simulink model "controller"  (R2019b)
settings: Solver=VariableStepAuto  StartTime=0.0  StopTime=10.0  RelTol=1e-3
undefined symbols (not defined in the file): maxPow1, maxPow2, maxPow3, maxTemp1, maxTemp2, maxTemp3, minTemp1, minTemp2, minTemp3, Pow1, Pow2, Pow3, Temp1, Temp2, Temp3
settings Model: Creator=wiart1  LastModifiedBy=tparis
settings DataIOCC: SaveFinalState=on  SaveOperatingPoint=on  SaveFormat=StructureWithTime  ReturnWorkspaceOutputs=off
settings DebuggingCC: ArithmeticOperatorsInVariantConditions=warning
settings SFSimCC: SimUseLocalCustomCode=off  CustomCodeUndefinedFunction=UseInterfaceOnly
settings RTWCC: RTWUseLocalCustomCode=off

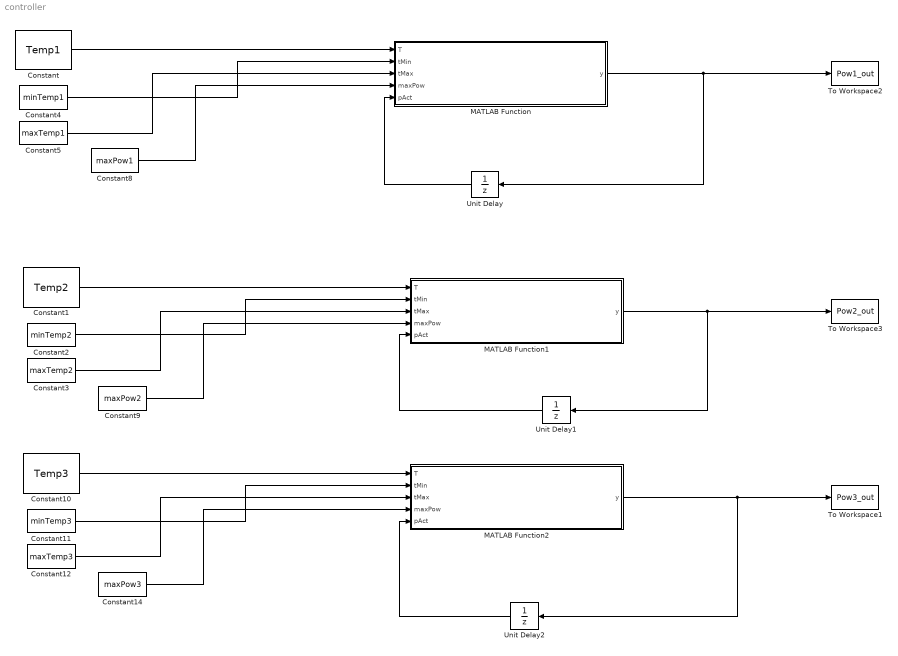
== system controller ==
  Constant : Constant  Value=Temp1
  Constant1 : Constant  Value=Temp2
  Constant10 : Constant  Value=Temp3
  Constant11 : Constant  Value=minTemp3
  Constant12 : Constant  Value=maxTemp3
  Constant14 : Constant  Value=maxPow3
  Constant2 : Constant  Value=minTemp2
  Constant3 : Constant  Value=maxTemp2
  Constant4 : Constant  Value=minTemp1
  Constant5 : Constant  Value=maxTemp1
  Constant8 : Constant  Value=maxPow1
  Constant9 : Constant  Value=maxPow2
  MATLAB Function : MATLAB Function  TreatAsAtomicUnit=on
  MATLAB Function1 : MATLAB Function  TreatAsAtomicUnit=on
  MATLAB Function2 : MATLAB Function  TreatAsAtomicUnit=on
  To Workspace1 : ToWorkspace  VariableName=Pow3_out  SaveFormat=Structure With Time  SampleTime=-1
  To Workspace2 : ToWorkspace  VariableName=Pow1_out  SaveFormat=Structure With Time  SampleTime=-1
  To Workspace3 : ToWorkspace  VariableName=Pow2_out  SaveFormat=Structure With Time  SampleTime=-1
  Unit Delay : UnitDelay  InitialCondition=Pow1  SampleTime=step  HasFrameUpgradeWarning=on
  Unit Delay1 : UnitDelay  InitialCondition=Pow2  SampleTime=step  HasFrameUpgradeWarning=on
  Unit Delay2 : UnitDelay  InitialCondition=Pow3  SampleTime=step  HasFrameUpgradeWarning=on
  wires:
  Constant/1 -> MATLAB Function/1(T)
  MATLAB Function/1(y) -> Unit Delay/1, To Workspace2/1
  Constant4/1 -> MATLAB Function/2(tMin)
  Constant5/1 -> MATLAB Function/3(tMax)
  Constant8/1 -> MATLAB Function/4(maxPow)
  Constant1/1 -> MATLAB Function1/1(T)
  MATLAB Function1/1(y) -> Unit Delay1/1, To Workspace3/1
  Constant9/1 -> MATLAB Function1/4(maxPow)
  Constant3/1 -> MATLAB Function1/3(tMax)
  Constant2/1 -> MATLAB Function1/2(tMin)
  Constant12/1 -> MATLAB Function2/3(tMax)
  Constant11/1 -> MATLAB Function2/2(tMin)
  Constant10/1 -> MATLAB Function2/1(T)
  Constant14/1 -> MATLAB Function2/4(maxPow)
  MATLAB Function2/1(y) -> Unit Delay2/1, To Workspace1/1
  Unit Delay/1 -> MATLAB Function/5(pAct)
  Unit Delay1/1 -> MATLAB Function1/5(pAct)
  Unit Delay2/1 -> MATLAB Function2/5(pAct)

== matlab function controller/MATLAB Function1 ==
  data: T input; y output; tMin input; tMax input; maxPow input; pAct input
function y = fcn(T, tMin, tMax, maxPow, pAct)
double p;
if T < tMin
    p = 0;
elseif  T > tMax
    p = maxPow;
else 
    p = pAct;
end

y = p;

== matlab function controller/MATLAB Function ==
  data: T input; y output; tMin input; tMax input; maxPow input; pAct input
function y = fcn(T, tMin, tMax, maxPow, pAct)
double p;
if T < tMin
    p = 0;
elseif  T > tMax
    p = maxPow;
else 
    p = pAct;
end

y = p;

== matlab function controller/MATLAB Function2 ==
  data: T input; y output; tMin input; tMax input; maxPow input; pAct input
function y = fcn(T, tMin, tMax, maxPow, pAct)
double p;
if T < tMin
    p = 0;
elseif  T > tMax
    p = maxPow;
else 
    p = pAct;
end

y = p;
